simulink model "Two_Level_Inverter_PLECS_lca"  (Simulink 7.8)
settings: Solver=FixedStepDiscrete  StartTime=0.0  StopTime=1  FixedStep=Ts_simulation  MaxStep=2e-3  RelTol=1e-3
PostLoadFcn:
  | Two_Level_Inverter_params;
InitFcn:
  | Two_Level_Inverter_params;
values from neighbouring files (symbols this model uses):
  Fc = 5000    [Two_Level_Inverter_params.m]
  Fout = 50    [Two_Level_Inverter_params.m]
  ModulationIndex = 0.95    [Two_Level_Inverter_params.m]
undefined symbols (not defined in the file or in its folder): DiscIntNeverNeededParam, plecs
settings Model: Creator=kris  LastModifiedBy=jonathanbouchard  ExtModeAutoUpdateStatusClock=off
settings DataIOCC: Refine=4
settings OptimizationCC: InitFltsAndDblsToZero=on
settings DebuggingCC: SaveWithParameterizedLinksMsg=none  FcnCallInpInsideContextMsg=Use local settings
settings CodeAppCC: CustomSymbolStrType=$N$R$M_T
settings GRTTargetCC: TargetFcnLib=ansi_tfl_tmw.mat  TargetFunctionLibrary=C89/C90 (ANSI)

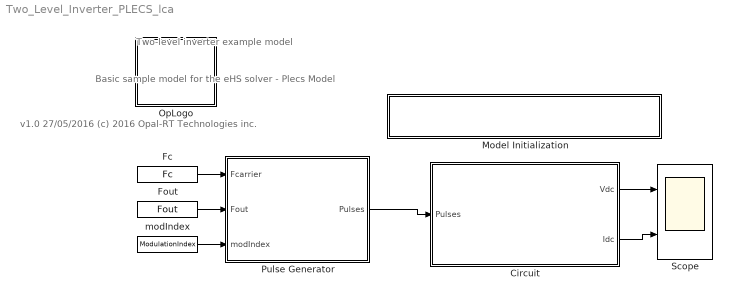
== system Two_Level_Inverter_PLECS_lca ==
  note: v1.0 27/05/2016
      | (c) 2016 Opal-RT Technologies inc.
  note: Two-level inverter example model
  note: Basic sample model for the eHS solver - Plecs Model
  Circuit : Subsystem  LoadFcn=plecs('sl', 200);  InitFcn=plecs('sl', 214);  StartFcn=plecs('sl', 208);  StopFcn=plecs('sl', 209);  mask(PlecsCircuit){PLECSData=<binary blob, 2600 chars, not shown>}
      mask prompts: PLECSData "PLECS Data (Do not delete or modify!)"
      mask init:
      | % PLACE CUSTOM INITIALIZATIONS ABOVE
      | % DO NOT REMOVE
      | plecs('sl', 215);
      | % DO NOT REMOVE
      settings: CopyFcn=plecs('sl', 203);  DeleteFcn=plecs('sl', 205);  UndoDeleteFcn=plecs('sl', 206);  PreSaveFcn=plecs('sl', 211);  PostSaveFcn=plecs('sl', 201);  NameChangeFcn=plecs('sl', 210);  DestroyFcn=plecs('sl', 207);  PreCopyFcn=plecs('sl', 216);  OpenFcn=plecs('sl', 202);  ErrorFcn=plerrorfcn
      mask Help: web(['file:///' fullfile(plecsdoc, 'creatingacircuit.html')])
      mask Display: disp('PLECS\nCircuit')
  Fc : Constant  Value=Fc
  Fout : Constant  Value=Fout
  Model Initialization : Subsystem  mask(Model Functions){InitFcnX=Two_Level_Inverter_params;, prel=off, posl=on, inif=on, strf=off}
      mask prompts: InitFcnX "Initialisation"; prel "Preload Function"; posl "PostLoad Function"; inif "InitFcn"; strf "StartFcn"
      mask init:
      | currentBlock = gcb;
      | root = bdroot(currentBlock);
      | 
      | if ~strcmp(get_param(root,'BlockDiagramType'),'library')
      |     if prel==1
      |         set_param(root, 'PreLoadFcn', InitFcnX);
      |     else
      |         set_param(root, 'PreLoadFcn', '');
      |     end
      |     if inif==1
      |         set_param(root, 'InitFcn', InitFcnX);
      |     else
      |         set_param(root, 'InitFcn', '');
      |     end
      |     if strf==1
      |         set_param(root, 'StartFcn', InitFcnX);
      |     else
      |         set_param(root, 'StartFcn', '');
      |     end
      |     if posl==1
      |         set_param(root, 'PostLoadFcn', InitFcnX);
      |     else
      |         set_param(root, 'PostLoadFcn', '');
      |     end
      | end
      | 
      | pos = get_param(currentBlock, 'Position');
      | width = pos(3) - pos(1); height = pos(4) - pos(2);
      | txt = [ upper(root) '\n' '- InitFcn. . . . . '  get_param(root, 'InitFcn') ];
      settings: CopyFcn=set_param(gcb,'LinkStatus','none')
      mask Display: text(5, height*0.5, txt, 'horizontalAlignment', 'left', 'verticalAlignment', 'middle') ;
  OpLogo : Subsystem
      mask Display:
      | opLogo = imread('LogoOpalRT.jpg');
      | image(opLogo(:,:,1:3));
  Pulse Generator : Subsystem
  Scope : Scope  NumInputPorts=2
      settings: YMin=-275000~-1  YMax=0~1  DataFormat=Array  MaxDataPoints=50000  Decimation=10
  modIndex : Constant  Value=ModulationIndex
  wires:
  Pulse Generator/1(Pulses) -> Circuit/1(Pulses)
  Fc/1 -> Pulse Generator/1(Fcarrier)
  Fout/1 -> Pulse Generator/2(Fout)
  modIndex/1 -> Pulse Generator/3(modIndex)
  Circuit/1(Vdc) -> Scope/1
  Circuit/2(Idc) -> Scope/2

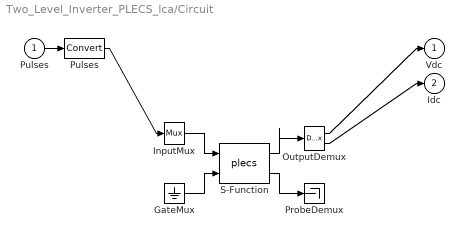
== system Two_Level_Inverter_PLECS_lca/Circuit ==
  Pulses : Inport  PortDimensions=3
  " GateMux " : Ground
  " InputMux " : Mux  Inputs=[ 3 ]
  " OutputDemux " : Demux  Outputs=[ 1 1 ]
  " ProbeDemux " : Terminator
  " Pulses " : DataTypeConversion  SaturateOnIntegerOverflow=on  RndMeth=Zero
  " S-Function " : S-Function  FunctionName=plecs  EnableBusSupport=off
  Vdc : Outport  PortDimensions=1
  Idc : Outport  Port=2  PortDimensions=1
  wires:
  " S-Function "/1 -> " OutputDemux "/1
  " InputMux "/1 -> " S-Function "/1
  " GateMux "/1 -> " S-Function "/2
  " S-Function "/2 -> " ProbeDemux "/1
  Pulses/1 -> " Pulses "/1
  " Pulses "/1 -> " InputMux "/1
  " OutputDemux "/1 -> Vdc/1
  " OutputDemux "/2 -> Idc/1

== system Two_Level_Inverter_PLECS_lca/Model Initialization ==

== system Two_Level_Inverter_PLECS_lca/OpLogo ==

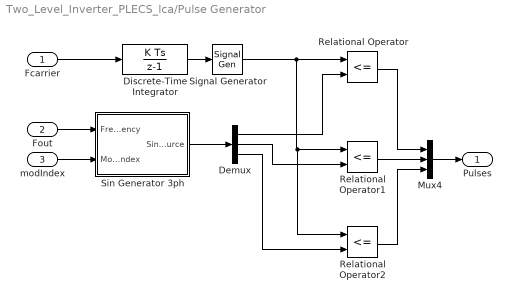
== system Two_Level_Inverter_PLECS_lca/Pulse Generator ==
  Fcarrier : Inport
  Fout : Inport  Port=2
  modIndex : Inport  Port=3
  Demux : Demux  Outputs=3
  Discrete-Time Integrator : DiscreteIntegrator  gainval=2*pi  SampleTime=-1  UpperSaturationLimit=2*pi  LowerSaturationLimit=-100*377  ICPrevOutput=DiscIntNeverNeededParam  ICPrevScaledInput=DiscIntNeverNeededParam
  Mux4 : Mux  Inputs=3
  Relational Operator : RelationalOperator  Operator=<=  OutDataTypeStr=boolean
  Relational Operator1 : RelationalOperator  Operator=<=  OutDataTypeStr=boolean
  Relational Operator2 : RelationalOperator  Operator=<=  OutDataTypeStr=boolean
  Signal Generator : SignalGenerator  WaveForm=sawtooth  TimeSource=Use external signal  Units=rad/sec
  Sin Generator 3ph : Subsystem
  Pulses : Outport
  wires:
  Demux/3 -> Relational Operator2/2
  Demux/2 -> Relational Operator1/2
  Demux/1 -> Relational Operator/2
  Sin Generator 3ph/1(Sin_Source) -> Demux/1
  Mux4/1 -> Pulses/1
  Signal Generator/1 -> Relational Operator2/1, Relational Operator1/1, Relational Operator/1
  Fout/1 -> Sin Generator 3ph/1(Frequency)
  modIndex/1 -> Sin Generator 3ph/2(ModulationIndex)
  Discrete-Time Integrator/1 -> Signal Generator/1
  Fcarrier/1 -> Discrete-Time Integrator/1
  Relational Operator/1 -> Mux4/1
  Relational Operator1/1 -> Mux4/2
  Relational Operator2/1 -> Mux4/3

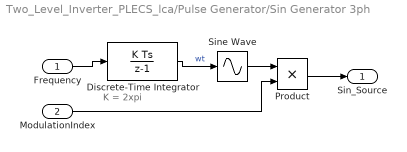
== system Two_Level_Inverter_PLECS_lca/Pulse Generator/Sin Generator 3ph ==
  note: K = 2xpi
  Frequency : Inport
  ModulationIndex : Inport  Port=2
  Discrete-Time Integrator : DiscreteIntegrator  gainval=2*pi  SampleTime=-1  UpperSaturationLimit=2*pi  LowerSaturationLimit=-100*377  ICPrevOutput=DiscIntNeverNeededParam  ICPrevScaledInput=DiscIntNeverNeededParam
  Product : Product
  Sine Wave : Sin  TimeSource=Use external signal  Phase=[0 -2*pi/3 2*pi/3]  SampleTime=0
  Sin_Source : Outport
  wires:
  Discrete-Time Integrator/1 -> Sine Wave/1  "wt"
  Frequency/1 -> Discrete-Time Integrator/1
  Sine Wave/1 -> Product/1
  Product/1 -> Sin_Source/1
  ModulationIndex/1 -> Product/2
